simulink model "lab1_variant1"  (R2024b)
settings: Solver=FixedStepDiscrete  StartTime=0  StopTime=30  FixedStep=dt  RelTol=1e-3
values from neighbouring files (symbols this model uses):
  B0 = 0    [part3.m]
  dt = 1    [part3.m]
  K = N    (= 17)    [part3.m]
  lambda0 = r(N)    [part3.m]
  mu0 = r(mod(N-2, group_size) + 1)    [part3.m]
undefined symbols (not defined in the file or in its folder): DiscIntNeverNeededParam
settings Model: Creator=SherOu  LastModifiedBy=SherOu

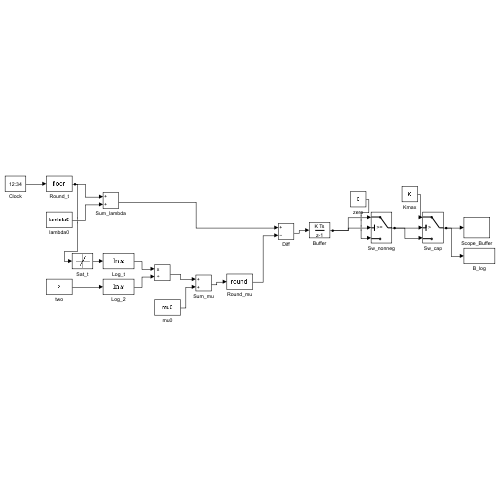
[thumbnail: Simulink's stored preview of the top-level diagram]
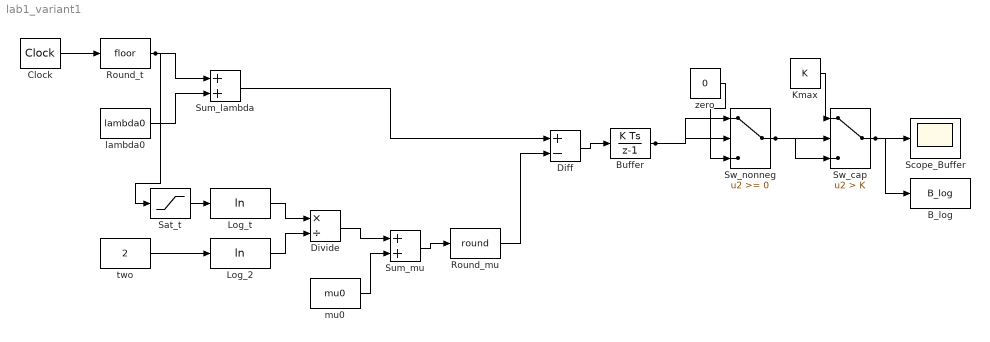
== system lab1_variant1 ==
  B_log : ToWorkspace  VariableName=B_log  SaveFormat=Timeseries  SampleTime=-1
  Buffer : DiscreteIntegrator  InitialCondition=B0  SampleTime=dt  ICPrevOutput=DiscIntNeverNeededParam  ICPrevScaledInput=DiscIntNeverNeededParam
  Clock : DigitalClock  SampleTime=dt
  Diff : Sum  Inputs=+-
  Divide : Product  Inputs=*/
  Kmax : Constant  Value=K
  Log_2 : Math  Operator=log
  Log_t : Math  Operator=log
  Round_mu : Rounding  Operator=round
  Round_t : Rounding
  Sat_t : Saturate  UpperLimit=inf  LowerLimit=1
  Scope_Buffer : Scope
  Sum_lambda : Sum
  Sum_mu : Sum
  Sw_cap : Switch  Criteria=u2 > Threshold  Threshold=K  SaturateOnIntegerOverflow=off  InputSameDT=off
  Sw_nonneg : Switch  SaturateOnIntegerOverflow=off  InputSameDT=off
  lambda0 : Constant  Value=lambda0
  mu0 : Constant  Value=mu0
  two : Constant  Value=2
  zero : Constant  Value=0
  wires:
  Clock/1 -> Round_t/1
  Round_t/1 -> Sum_lambda/1, Sat_t/1
  lambda0/1 -> Sum_lambda/2
  Sat_t/1 -> Log_t/1
  two/1 -> Log_2/1
  Log_t/1 -> Divide/1
  Log_2/1 -> Divide/2
  Divide/1 -> Sum_mu/1
  mu0/1 -> Sum_mu/2
  Sum_mu/1 -> Round_mu/1
  Sum_lambda/1 -> Diff/1
  Round_mu/1 -> Diff/2
  Diff/1 -> Buffer/1
  Buffer/1 -> Sw_nonneg/2, Sw_nonneg/1
  zero/1 -> Sw_nonneg/3
  Sw_nonneg/1 -> Sw_cap/2, Sw_cap/3
  Kmax/1 -> Sw_cap/1
  Sw_cap/1 -> Scope_Buffer/1, B_log/1
